simulink model "Part_3_3_figure"  (R2018a)
settings: Solver=VariableStepAuto  StartTime=0.0  StopTime=1  MaxStep=1e-6  RelTol=1e-3
libraries: powerlib x16, peRmsMeasurement x2
settings Model: Creator=Ekin Su Saçın  LastModifiedBy=Ekin Su Saçın

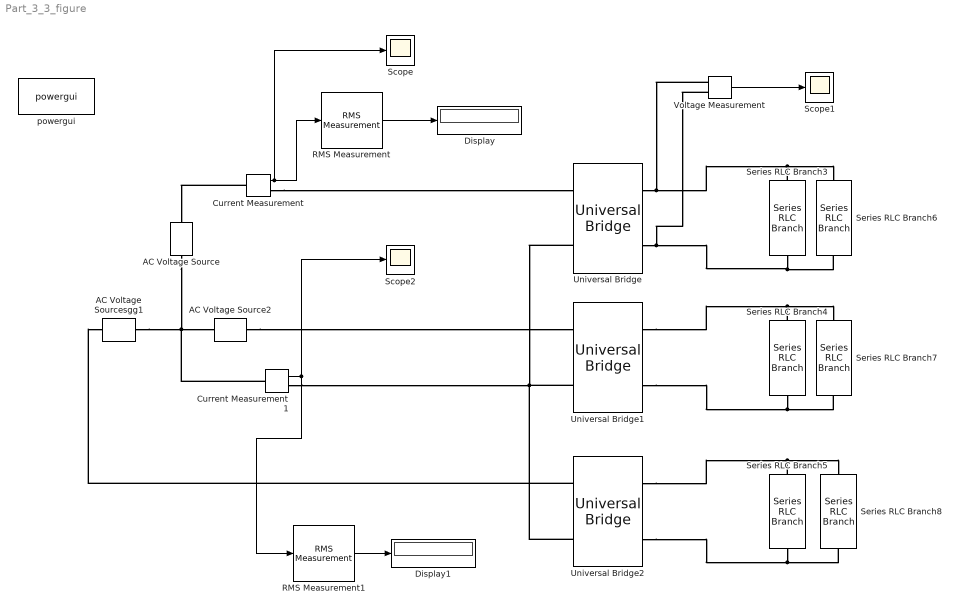
== system Part_3_3_figure ==
  AC Voltage Source : powerlib/Electrical Sources/AC Voltage Source  Amplitude=200  Phase=0  Frequency=50  SampleTime=0  Measurements=Voltage  BusType=swing  Pref=10e3  Qref=0  Qmin=-inf  Qmax=+inf
  AC Voltage Source2 : powerlib/Electrical Sources/AC Voltage Source  Amplitude=200  Phase=-120  Frequency=50  SampleTime=0  Measurements=Voltage  BusType=swing  Pref=10e3  Qref=0  Qmin=-inf  Qmax=+inf
  AC Voltage Sourcesgg1 : powerlib/Electrical Sources/AC Voltage Source  Amplitude=200  Phase=120  Frequency=50  SampleTime=0  Measurements=Voltage  BusType=swing  Pref=10e3  Qref=0  Qmin=-inf  Qmax=+inf
  Current Measurement : powerlib/Measurements/Current Measurement  PhasorSimulation=off  OutputType=Complex  PSBequivalent=0
  Current Measurement1 : powerlib/Measurements/Current Measurement  PhasorSimulation=off  OutputType=Complex  PSBequivalent=0
  Display : Display
  Display1 : Display
  RMS Measurement : peRmsMeasurement/RMS Measurement  OverrideUsingVariant=Total  F=60  SpecifyHarmonics=off  K=[0 1 2]  Ts=0
  RMS Measurement1 : peRmsMeasurement/RMS Measurement  OverrideUsingVariant=Total  F=60  SpecifyHarmonics=off  K=[0 1 2]  Ts=0
  Scope : Scope
  Scope1 : Scope
  Scope2 : Scope
  Series RLC Branch3 : powerlib/Elements/Series RLC Branch  LConnTagsString=__new0  RConnTagsString=__new0  BranchType=R  Resistance=200  Inductance=1e-3  SetiL0=off  InitialCurrent=0  Capacitance=1e-6  Setx0=off  InitialVoltage=0  Measurements=Branch voltage
  Series RLC Branch4 : powerlib/Elements/Series RLC Branch  LConnTagsString=__new0  RConnTagsString=__new0  BranchType=R  Resistance=200  Inductance=1e-3  SetiL0=off  InitialCurrent=0  Capacitance=1e-6  Setx0=off  InitialVoltage=0  Measurements=None
  Series RLC Branch5 : powerlib/Elements/Series RLC Branch  LConnTagsString=__new0  RConnTagsString=__new0  BranchType=R  Resistance=200  Inductance=1e-3  SetiL0=off  InitialCurrent=0  Capacitance=1e-6  Setx0=off  InitialVoltage=0  Measurements=None
  Series RLC Branch6 : powerlib/Elements/Series RLC Branch  LConnTagsString=__new0  RConnTagsString=__new0  BranchType=C  Resistance=200  Inductance=1e-3  SetiL0=off  InitialCurrent=0  Capacitance=470*1e-6  Setx0=off  InitialVoltage=0  Measurements=Branch voltage
  Series RLC Branch7 : powerlib/Elements/Series RLC Branch  LConnTagsString=__new0  RConnTagsString=__new0  BranchType=C  Resistance=200  Inductance=1e-3  SetiL0=off  InitialCurrent=0  Capacitance=470*1e-6  Setx0=off  InitialVoltage=0  Measurements=None
  Series RLC Branch8 : powerlib/Elements/Series RLC Branch  LConnTagsString=__new0  RConnTagsString=__new0  BranchType=C  Resistance=200  Inductance=1e-3  SetiL0=off  InitialCurrent=0  Capacitance=470*1e-6  Setx0=off  InitialVoltage=0  Measurements=None
  Universal Bridge : powerlib/Power Electronics/Universal Bridge  Arms=2  SnubberResistance=1e5  SnubberCapacitance=inf  Device=Diodes  Ron=1e-3  Lon=0  ForwardVoltages="[  0  0  ]"  ForwardVoltage=0  GTOparameters=[ 10e-6 , 20e-6 ]  IGBTparameters=[ 1e-6 , 2e-6 ]  Measurements=All voltages and currents  Measurements_2=None  converterType=Rectifier
  Universal Bridge1 : powerlib/Power Electronics/Universal Bridge  Arms=2  SnubberResistance=1e5  SnubberCapacitance=inf  Device=Diodes  Ron=1e-3  Lon=0  ForwardVoltages="[  0  0  ]"  ForwardVoltage=0  GTOparameters=[ 10e-6 , 20e-6 ]  IGBTparameters=[ 1e-6 , 2e-6 ]  Measurements=None  Measurements_2=None  converterType=Rectifier
  Universal Bridge2 : powerlib/Power Electronics/Universal Bridge  Arms=2  SnubberResistance=1e5  SnubberCapacitance=inf  Device=Diodes  Ron=1e-3  Lon=0  ForwardVoltages="[  0  0  ]"  ForwardVoltage=0  GTOparameters=[ 10e-6 , 20e-6 ]  IGBTparameters=[ 1e-6 , 2e-6 ]  Measurements=None  Measurements_2=None  converterType=Rectifier
  Voltage Measurement : powerlib/Measurements/Voltage Measurement  PhasorSimulation=off  OutputType=Complex  PSBequivalent=0
  powergui : powerlib/powergui  Priority=1  SimulationMode=Continuous  SampleTime=50e-6  frequency=60  Iterations=50  frequencyindice=50  Pbase=100e6  ErrMax=1e-4  UnitsV=kV  UnitsW=MW  buscounter=0  FunctionMessages=off  echomessages=off  EnableUseOfTLC=off  CurrentSourceSwitches=off  DisableSnubberDevices=off  DisableRonSwitches=off  DisableVfSwitches=off  DisplayEquations=off  SolverType=Tustin/Backward Euler (TBE)  Interpol=off  ExternalGateDelay=off  methode=off  Ts=100  x0status=blocks  SPID=on  SwTol=0  HookPort=off  RestoreLinks=warning  ResistiveCurrentMeasurement=off  Frange=[0:2:500]  Ylog=off  Xlog=on  ShowGrid=off  save=off  variable=ZData  structure=0  ZoomFFT=off  StartTime=0.0  cycles=1  DisplayStyle=1  fundamental=60  FreqAxis=off  MaxFrequency=1000  frequencyindicesteady=1  RmsSteady=1  display=off
  wires:
  Voltage Measurement/1 -> Scope1/1
  Current Measurement1/1 -> Scope2/1, RMS Measurement1/1
  RMS Measurement/1 -> Display/1
  RMS Measurement1/1 -> Display1/1
  Current Measurement/1 -> Scope/1, RMS Measurement/1
  connections:
  Series RLC Branch3/LConn1 -- Voltage Measurement/LConn1 -- Universal Bridge/RConn1 -- Series RLC Branch6/LConn1
  Series RLC Branch3/RConn1 -- Voltage Measurement/LConn2 -- Universal Bridge/RConn2 -- Series RLC Branch6/RConn1
  Series RLC Branch4/LConn1 -- Universal Bridge1/RConn1 -- Series RLC Branch7/LConn1
  Series RLC Branch4/RConn1 -- Universal Bridge1/RConn2 -- Series RLC Branch7/RConn1
  Series RLC Branch5/LConn1 -- Universal Bridge2/RConn1 -- Series RLC Branch8/LConn1
  Series RLC Branch5/RConn1 -- Universal Bridge2/RConn2 -- Series RLC Branch8/RConn1
  Current Measurement/RConn1 -- Universal Bridge/LConn1
  AC Voltage Source2/RConn1 -- Universal Bridge1/LConn1
  Universal Bridge1/LConn2 -- Universal Bridge2/LConn2 -- Current Measurement1/RConn1 -- Universal Bridge/LConn2
  Universal Bridge2/LConn1 -- AC Voltage Sourcesgg1/RConn1
  Current Measurement/LConn1 -- AC Voltage Source/RConn1
  AC Voltage Sourcesgg1/LConn1 -- Current Measurement1/LConn1 -- AC Voltage Source/LConn1 -- AC Voltage Source2/LConn1
